simulink library "INT_AccPed_DoCoordOut"  (R2016b)
settings: Solver=VariableStepAuto  StartTime=0.0  StopTime=10.0  RelTol=1e-3
settings Model: Creator=bianxuyin  LastModifiedBy=bianxuyin

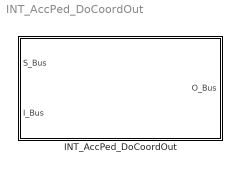
== system INT_AccPed_DoCoordOut ==
  INT_AccPed_DoCoordOut : Subsystem

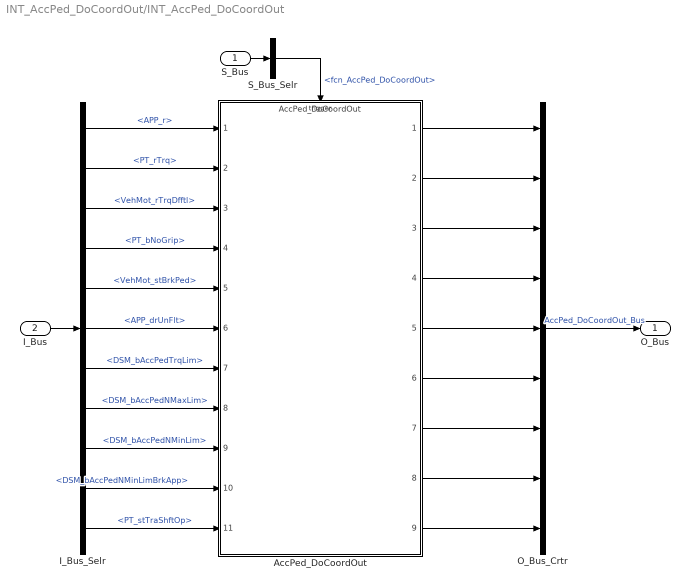
== system INT_AccPed_DoCoordOut/INT_AccPed_DoCoordOut ==
  S_Bus : Inport
  I_Bus : Inport  Port=2
  AccPed_DoCoordOut : ModelReference  ModelNameDialog=AccPed_DoCoordOut  SimulationMode=Normal  ModelReferenceVersion=1.28  TriggerPortName=function  TriggerPortTriggerType=function-call  TriggerPortStatesWhenEnabling=held
  I_Bus_Selr : BusSelector  OutputSignals=APP_r,PT_rTrq,VehMot_rTrqDfftl,PT_bNoGrip,VehMot_stBrkPed,APP_drUnFlt,DSM_bAccPedTrqLim,DSM_bAccPedNMaxLim,DSM_bAccPedNMinLim,DSM_bAccPedNMinLimBrkApp,PT_stTraShftOp
  O_Bus_Crtr : BusCreator  Inputs=9
  S_Bus_Selr : BusSelector  OutputSignals=fcn_AccPed_DoCoordOut
  O_Bus : Outport
  wires:
  S_Bus_Selr/1 -> AccPed_DoCoordOut/Trigger  "<fcn_AccPed_DoCoordOut>"
  S_Bus/1 -> S_Bus_Selr/1
  I_Bus/1 -> I_Bus_Selr/1
  I_Bus_Selr/1 -> AccPed_DoCoordOut/1  "<APP_r>"
  I_Bus_Selr/2 -> AccPed_DoCoordOut/2  "<PT_rTrq>"
  I_Bus_Selr/3 -> AccPed_DoCoordOut/3  "<VehMot_rTrqDfftl>"
  I_Bus_Selr/4 -> AccPed_DoCoordOut/4  "<PT_bNoGrip>"
  I_Bus_Selr/5 -> AccPed_DoCoordOut/5  "<VehMot_stBrkPed>"
  I_Bus_Selr/6 -> AccPed_DoCoordOut/6  "<APP_drUnFlt>"
  I_Bus_Selr/7 -> AccPed_DoCoordOut/7  "<DSM_bAccPedTrqLim>"
  I_Bus_Selr/8 -> AccPed_DoCoordOut/8  "<DSM_bAccPedNMaxLim>"
  I_Bus_Selr/9 -> AccPed_DoCoordOut/9  "<DSM_bAccPedNMinLim>"
  I_Bus_Selr/10 -> AccPed_DoCoordOut/10  "<DSM_bAccPedNMinLimBrkApp>"
  I_Bus_Selr/11 -> AccPed_DoCoordOut/11  "<PT_stTraShftOp>"
  O_Bus_Crtr/1 -> O_Bus/1  "AccPed_DoCoordOut_Bus"
  AccPed_DoCoordOut/1 -> O_Bus_Crtr/1
  AccPed_DoCoordOut/2 -> O_Bus_Crtr/2
  AccPed_DoCoordOut/3 -> O_Bus_Crtr/3
  AccPed_DoCoordOut/4 -> O_Bus_Crtr/4
  AccPed_DoCoordOut/5 -> O_Bus_Crtr/5
  AccPed_DoCoordOut/6 -> O_Bus_Crtr/6
  AccPed_DoCoordOut/7 -> O_Bus_Crtr/7
  AccPed_DoCoordOut/8 -> O_Bus_Crtr/8
  AccPed_DoCoordOut/9 -> O_Bus_Crtr/9
